simulink model "SimulinlThing"  (R2016b)
settings: Solver=ode4  StartTime=0.0  StopTime=T  FixedStep=dt  RelTol=1e-3
values from neighbouring files (symbols this model uses):
  A = [0,1,0,0 ... (first row only)    [LabScript.m]
  B = [0;1/J1;0;0]    [LabScript.m]
  C = [0,0,0,1]    [LabScript.m]
  D = [0]    [LabScript.m]
settings Model: Creator=melabuser  LastModifiedBy=melabuser

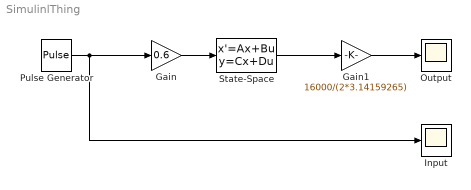
== system SimulinlThing ==
  Gain : Gain  Gain=0.6
  Gain1 : Gain  Gain=16000/(2*3.14159265)
  Input : Scope
  Output : Scope
  Pulse Generator : DiscretePulseGenerator  PulseType=Time based  Amplitude=0.5  Period=1.325  PulseWidth=7.55
  State-Space : StateSpace  A=A  B=B  C=C  D=D  X0=0
  wires:
  Pulse Generator/1 -> Input/1, Gain/1
  Gain/1 -> State-Space/1
  State-Space/1 -> Gain1/1
  Gain1/1 -> Output/1
